simulink model "MassTransfer"  (R2023a)
settings: Solver=ode4  StartTime=0.0  StopTime=7540  FixedStep=Delta  RelTol=1e-3
values from neighbouring files (symbols this model uses):
  C2Ini = 1.6    [MassTransferModelData.m]
  C3Ini = 0    [MassTransferModelData.m]
  C4Ini = 0    [MassTransferModelData.m]
  C5Ini = 1.6    [MassTransferModelData.m]
  Delta = 5    [MassTransferModelData.m]
  F = 96485    [MassTransferModelData.m]
  NCells = 120    [MassTransferModelData.m]
  VCell = 0.4968    [MassTransferModelData.m]
  VTank = 500    [MassTransferModelData.m]
  z = 1    [MassTransferModelData.m]
undefined symbols (not defined in the file or in its folder): DiscIntNeverNeededParam
(part 3 of 3)

== matlab function MassTransfer/QF tests1/Analitical/C3Cell/MATLAB Function ==
  data: QCell input; CCell output; CTank input; CCellAnt input; VCell input; It input; F input; Z input; Sign input; Delta input
function CCell = fcn(QCell, CTank, CCellAnt, VCell, It, F, Z, Sign, Delta)
    K1 = QCell*(1/(VCell/2));
    K2 = (1/(VCell/2))*(1/(Z*F));
    CCell = (K1*Delta*CTank + Sign*K2*Delta*It + CCellAnt)/(1+K1*Delta);
end

== matlab function MassTransfer/QF tests/Analitical/C2Cell/MATLAB Function ==
  data: QCell input; CCell output; CTank input; CCellAnt input; VCell input; It input; F input; Z input; Sign input; Delta input
function CCell = fcn(QCell, CTank, CCellAnt, VCell, It, F, Z, Sign, Delta)
    K1 = QCell*(1/(VCell/2));
    K2 = (1/(VCell/2))*(1/(Z*F));
    CCell = (K1*Delta*CTank + Sign*K2*Delta*It + CCellAnt)/(1+K1*Delta);
end

== matlab function MassTransfer/QF tests1/Analitical/C3Tank/MATLAB Function ==
  data: Q input; CTank output; CCell input; CTankAnt input; VTank input; Delta input
function CTank = fcn(Q, CCell, CTankAnt, VTank, Delta)
    K3 = Q/VTank;
    CTank = (CCell*K3*Delta + CTankAnt)/(1+K3*Delta);
end

== matlab function MassTransfer/QF tests1/Analitical/C4Cell/MATLAB Function ==
  data: QCell input; CCell output; CTank input; CCellAnt input; VCell input; It input; F input; Z input; Sign input; Delta input
function CCell = fcn(QCell, CTank, CCellAnt, VCell, It, F, Z, Sign, Delta)
    K1 = QCell*(1/(VCell/2));
    K2 = (1/(VCell/2))*(1/(Z*F));
    CCell = (K1*Delta*CTank + Sign*K2*Delta*It + CCellAnt)/(1+K1*Delta);
end

== matlab function MassTransfer/QF tests1/Analitical/C4Tank/MATLAB Function ==
  data: Q input; CTank output; CCell input; CTankAnt input; VTank input; Delta input
function CTank = fcn(Q, CCell, CTankAnt, VTank, Delta)
    K3 = Q/VTank;
    CTank = (CCell*K3*Delta + CTankAnt)/(1+K3*Delta);
end

== matlab function MassTransfer/QF tests1/Analitical/C5Cell/MATLAB Function ==
  data: QCell input; CCell output; CTank input; CCellAnt input; VCell input; It input; F input; Z input; Sign input; Delta input
function CCell = fcn(QCell, CTank, CCellAnt, VCell, It, F, Z, Sign, Delta)
    K1 = QCell*(1/(VCell/2));
    K2 = (1/(VCell/2))*(1/(Z*F));
    CCell = (K1*Delta*CTank + Sign*K2*Delta*It + CCellAnt)/(1+K1*Delta);
end

== matlab function MassTransfer/QF tests1/Analitical/C5Tank/MATLAB Function ==
  data: Q input; CTank output; CCell input; CTankAnt input; VTank input; Delta input
function CTank = fcn(Q, CCell, CTankAnt, VTank, Delta)
    K3 = Q/VTank;
    CTank = (CCell*K3*Delta + CTankAnt)/(1+K3*Delta);
end

== matlab function MassTransfer/QF tests3/Analitical/C2Cell/MATLAB Function ==
  data: QCell input; CCell output; CTank input; CCellAnt input; VCell input; It input; F input; Z input; Sign input; Delta input
function CCell = fcn(QCell, CTank, CCellAnt, VCell, It, F, Z, Sign, Delta)
    K1 = QCell*(1/(VCell/2));
    K2 = (1/(VCell/2))*(1/(Z*F));
    CCell = (K1*Delta*CTank + Sign*K2*Delta*It + CCellAnt)/(1+K1*Delta);
end

== matlab function MassTransfer/QF tests1/Flow calculation anal/MATLAB Function ==
  data: C2 input; QCell output; C3 input; C4 input; C5 input; I input; F input; QF input
function QCell = fcn(C2, C3, C4, C5, I, F, QF)
    if I > 0
        QCell = QF*abs(I)/(F*(C2+C5)/2);
    else
        QCell = QF*abs(I)/(F*(C3+C4)/2);
    end
end

== matlab function MassTransfer/Concentration comparator/MATLAB Function ==
  data: C2 input; Eoc output; C3 input; C4 input; C5 input
function Eoc = fcn(C2, C3, C4, C5)
    Eoc = 1.4 + 293*8.314/(96485*1)*log(C2*C5/(C3*C4));
end

== matlab function MassTransfer/Concentration comparator/MATLAB Function1 ==
  data: C2 input; Eoc output; C3 input; C4 input; C5 input
function Eoc = fcn(C2, C3, C4, C5)
    Eoc = 1.4 + 293*8.314/(96485*1)*log(C2*C5/(C3*C4));
end

== matlab function MassTransfer/QF tests3/Analitical/C2Tank/MATLAB Function ==
  data: Q input; CTank output; CCell input; CTankAnt input; VTank input; Delta input
function CTank = fcn(Q, CCell, CTankAnt, VTank, Delta)
    K3 = Q/VTank;
    CTank = (CCell*K3*Delta + CTankAnt)/(1+K3*Delta);
end

== matlab function MassTransfer/QF tests3/Analitical/C3Cell/MATLAB Function ==
  data: QCell input; CCell output; CTank input; CCellAnt input; VCell input; It input; F input; Z input; Sign input; Delta input
function CCell = fcn(QCell, CTank, CCellAnt, VCell, It, F, Z, Sign, Delta)
    K1 = QCell*(1/(VCell/2));
    K2 = (1/(VCell/2))*(1/(Z*F));
    CCell = (K1*Delta*CTank + Sign*K2*Delta*It + CCellAnt)/(1+K1*Delta);
end

== matlab function MassTransfer/QF tests3/Analitical/C3Tank/MATLAB Function ==
  data: Q input; CTank output; CCell input; CTankAnt input; VTank input; Delta input
function CTank = fcn(Q, CCell, CTankAnt, VTank, Delta)
    K3 = Q/VTank;
    CTank = (CCell*K3*Delta + CTankAnt)/(1+K3*Delta);
end

== matlab function MassTransfer/QF tests3/Analitical/C4Cell/MATLAB Function ==
  data: QCell input; CCell output; CTank input; CCellAnt input; VCell input; It input; F input; Z input; Sign input; Delta input
function CCell = fcn(QCell, CTank, CCellAnt, VCell, It, F, Z, Sign, Delta)
    K1 = QCell*(1/(VCell/2));
    K2 = (1/(VCell/2))*(1/(Z*F));
    CCell = (K1*Delta*CTank + Sign*K2*Delta*It + CCellAnt)/(1+K1*Delta);
end

== matlab function MassTransfer/QF tests/Analitical/C3Cell/MATLAB Function ==
  data: QCell input; CCell output; CTank input; CCellAnt input; VCell input; It input; F input; Z input; Sign input; Delta input
function CCell = fcn(QCell, CTank, CCellAnt, VCell, It, F, Z, Sign, Delta)
    K1 = QCell*(1/(VCell/2));
    K2 = (1/(VCell/2))*(1/(Z*F));
    CCell = (K1*Delta*CTank + Sign*K2*Delta*It + CCellAnt)/(1+K1*Delta);
end

== matlab function MassTransfer/QF tests3/Analitical/C4Tank/MATLAB Function ==
  data: Q input; CTank output; CCell input; CTankAnt input; VTank input; Delta input
function CTank = fcn(Q, CCell, CTankAnt, VTank, Delta)
    K3 = Q/VTank;
    CTank = (CCell*K3*Delta + CTankAnt)/(1+K3*Delta);
end

== matlab function MassTransfer/QF tests3/Analitical/C5Cell/MATLAB Function ==
  data: QCell input; CCell output; CTank input; CCellAnt input; VCell input; It input; F input; Z input; Sign input; Delta input
function CCell = fcn(QCell, CTank, CCellAnt, VCell, It, F, Z, Sign, Delta)
    K1 = QCell*(1/(VCell/2));
    K2 = (1/(VCell/2))*(1/(Z*F));
    CCell = (K1*Delta*CTank + Sign*K2*Delta*It + CCellAnt)/(1+K1*Delta);
end

== matlab function MassTransfer/Library block sustituyendo I//(zF) en las ecuaciones/QF tests2/Flow calculation anal/MATLAB Function ==
  data: C2 input; QCell output; C3 input; C4 input; C5 input; I input; F input; QF input
function QCell = fcn(C2, C3, C4, C5, I, F, QF)
    if I > 0
        QCell = QF*abs(I)/(F*(C2+C5)/2);
    else
        QCell = QF*abs(I)/(F*(C3+C4)/2);
    end
end

== matlab function MassTransfer/QF tests3/Analitical/C5Tank/MATLAB Function ==
  data: Q input; CTank output; CCell input; CTankAnt input; VTank input; Delta input
function CTank = fcn(Q, CCell, CTankAnt, VTank, Delta)
    K3 = Q/VTank;
    CTank = (CCell*K3*Delta + CTankAnt)/(1+K3*Delta);
end

== matlab function MassTransfer/QF tests3/Flow calculation anal/MATLAB Function ==
  data: C2 input; QCell output; C3 input; C4 input; C5 input; I input; F input; QF input
function QCell = fcn(C2, C3, C4, C5, I, F, QF)
    if I > 0
        QCell = QF*abs(I)/(F*(C2+C5)/2);
    else
        QCell = QF*abs(I)/(F*(C3+C4)/2);
    end
end

== matlab function MassTransfer/Concentration comparator1/MATLAB Function ==
  data: C2 input; Eoc output; C3 input; C4 input; C5 input
function Eoc = fcn(C2, C3, C4, C5)
    Eoc = 1.4 + 293*8.314/(96485*1)*log(C2*C5/(C3*C4));
end

== matlab function MassTransfer/Concentration comparator1/MATLAB Function1 ==
  data: C2 input; Eoc output; C3 input; C4 input; C5 input
function Eoc = fcn(C2, C3, C4, C5)
    Eoc = 1.4 + 293*8.314/(96485*1)*log(C2*C5/(C3*C4));
end

== matlab function MassTransfer/QF tests4/Flow calculation anal/MATLAB Function ==
  data: C2 input; QCell output; C3 input; C4 input; C5 input; I input; F input; QF input
function QCell = fcn(C2, C3, C4, C5, I, F, QF)
    if I > 0
        QCell = QF*abs(I)/(F*(C2+C5)/2);
    else
        QCell = QF*abs(I)/(F*(C3+C4)/2);
    end
end

== matlab function MassTransfer/QF tests5/Flow calculation anal/MATLAB Function ==
  data: C2 input; QCell output; C3 input; C4 input; C5 input; I input; F input; QF input
function QCell = fcn(C2, C3, C4, C5, I, F, QF)
    if I > 0
        QCell = QF*abs(I)/(F*(C2+C5)/2);
    else
        QCell = QF*abs(I)/(F*(C3+C4)/2);
    end
end

== matlab function MassTransfer/QF tests/Analitical/C4Cell/MATLAB Function ==
  data: QCell input; CCell output; CTank input; CCellAnt input; VCell input; It input; F input; Z input; Sign input; Delta input
function CCell = fcn(QCell, CTank, CCellAnt, VCell, It, F, Z, Sign, Delta)
    K1 = QCell*(1/(VCell/2));
    K2 = (1/(VCell/2))*(1/(Z*F));
    CCell = (K1*Delta*CTank + Sign*K2*Delta*It + CCellAnt)/(1+K1*Delta);
end

== matlab function MassTransfer/QF tests/Analitical/C5Cell/MATLAB Function ==
  data: QCell input; CCell output; CTank input; CCellAnt input; VCell input; It input; F input; Z input; Sign input; Delta input
function CCell = fcn(QCell, CTank, CCellAnt, VCell, It, F, Z, Sign, Delta)
    K1 = QCell*(1/(VCell/2));
    K2 = (1/(VCell/2))*(1/(Z*F));
    CCell = (K1*Delta*CTank + Sign*K2*Delta*It + CCellAnt)/(1+K1*Delta);
end

== matlab function MassTransfer/QF tests/Analitical/C2Tank/MATLAB Function ==
  data: Q input; CTank output; CCell input; CTankAnt input; VTank input; Delta input
function CTank = fcn(Q, CCell, CTankAnt, VTank, Delta)
    K3 = Q/VTank;
    CTank = (CCell*K3*Delta + CTankAnt)/(1+K3*Delta);
end
